simulink model "FlameAnalysis"  (R2015b)
settings: Solver=ode45  SolverMode=SingleTasking  StartTime=0.0  StopTime=1000  RelTol=1e-3
PreLoadFcn:
  | fprintf('loading now...\n')
PostLoadFcn:
  | model_name = gcs;
  | video_player_name=[model_name, '/From Multimedia File'];
  | video_path=get_param(video_player_name,'inputFileName');
  | model_path= get_param(model_name,'filename');
  | i=findstr('\',model_path);
  | 
  | if(~exist(video_path))
  |      video_path2=[model_path(1:i(end))  video_path(findstr('Video',video_path):end)];
  | 
  |      if(exist(video_path2))
  |           set_param(video_player_name,'inputFileName',video_path2);
  |      else
  |           j=findstr('\',video_path);
  |           video_path2=[model_path(1:i(end))  'Videos\' video_path(j(end)+1:end)];
  |           if(exist(video_path2))
  |                set_param(video_player_name,'inputFileName',video_path2);
  |           else
  |                avifiles=dir('videos\*.avi')
  |                set_param(video_player_name,'inputFileName',[model_path(1:i(end))  'Videos\'   avifiles(1).name]);
  |           end
  | 
  |      end
  | end
InitFcn:
  | clc
  | clear
  | global  t position wide dz_dt d2z_dt2 d3z_dt3 Af As dA_dt filePath Su_ Su alfa Karlovitz threshold model_name bords tWalls sheet model_path simulating numPointsAnalysis
  | simulating=true;
  | model_name = gcs;
  | model_path = [model_name, '/Edit Parameters'];
  | tbf = str2num(get_param(model_path,'tbf'));
  | ppcm= str2num(get_param(model_path,'ppcm'));
  | p2e= str2num(get_param(model_path,'p2e'));
  | 
  | nframes0= str2num(get_param(model_path,'nframes0'));
  | alfa= str2num(get_param(model_path,'alfa'));
  | fff= str2num(get_param(model_path,'fff'));
  | 
  | if((size(fff,2)~=1) & (size(fff,2)~=2))
  |     error('The flame front fraction must be scalar or 1x2-array');
  | end
  | order=str2num(get_param(model_path,'order'));
  | numberOfPoints=str2num(get_param(model_path,'numberOfPoints'));
  | orderAnalysis=str2num(get_param(model_path,'orderAnalysis'));
  | numPointsAnalysis=str2num(get_param(model_path,'numPointsAnalysis'));
  | uselog=str2num(get_param(model_path,'uselog'));
  | 
  | 
  | save2xls= strcmp('on',get_param(model_path,'save2xls'));
  | saveVideo= strcmp('on',get_param(model_path,'saveVideo'));
  | cfs= strcmp('on',get_param(model_path,'cfs'));
  | c3dv= strcmp('on',get_param(model_path,'c3dv'));
  | 
  | 
  | if(strcmp(get_param(model_path,'bge'),'Temporal Median Estimator'))
  |      bge=1;
  | elseif (strcmp(get_param(model_path,'bge'),'Temporal Median'))
  |     bge=2;
  |     bkgnd{1}=[gcs '/Background Estimator/Decomposing Red Movement/BG1/Temporal Median/Temporal Median'];
  |     bkgnd{2}=[gcs '/Background Estimator/Decomposing Green Movement/BG1/Temporal Median/Temporal Median'];
  |     bkgnd{3}=[gcs '/Background Estimator/Decomposing Blue Movement/BG1/Temporal Median/Temporal Median'];
  | 
  |     nframes0=max(nframes0,1);
  |     set_param([gcs '/Edit Parameters/'],'nframes0',num2str(nframes0));
  |     for i=1:3
  |         set_param(bkgnd{i}, 'tw', num2str(nframes0));
  |     end
  | else
  |     bge=3;
  | end
  | 
  | 
  | 
  | switch(get_param(model_path,'aprox_type'))
  |      case 'Profile'
  |            aprox_type=1;
  |            sheet='Profile';
  |      case 'Paraboloid (moving base)'
  |            aprox_type=2;
  |            sheet='Paraboloid';
  |      case 'Paraboloid(fixed base)'
  |            aprox_type=3;
  |            sheet='ParaboloidFB';
  |      case 'Spheroid'
  | ... (+19 lines)
StopFcn:
  | global editing  simulating
  | simulating = true;
  | try
  |       closeFunction
  | catch err
  |       simulating=false;
  |       err
  | end
  |   simulating=false;
model workspace (MATLAB code in the model file):
  | line_row =  22;
values from neighbouring files (symbols this model uses):
  m = size(BW,1)    [flameFront.m]    (also in putCircles.m = (y(i+1)-y(i))./(x(i+1)-x(i)))
  n = n(n==size(num,2)/4)    [averageOfVideos.m]    (also in countFramesOfVideo.m = 1; putCircles.m = length(y))
  vector = cast([row, col],'double')    [flameFront.m]
undefined symbols (not defined in the file or in its folder): strel
libraries: simulink x27, visionstatistics x14, visionconversions x9, visiontextngfix x9, visionmorphops x7, dspvision x4, visionsinks x2, visiongeotforms x1
(part 3 of 3)

== matlab function FlameAnalysis/Flame Front Estimation/Embedded MATLAB Function ==
  data: BW input; BBox input; Y output size=[2 (size(BW,1)*2 + size(BW,2)*2)*50] [0..1000000]; L output size=[1 size(BW,1)*100 ] [0..1000000]; fraction input; y_electrodes input; profile input; newBW output size=size(BW)
%Function that analyses a boolean image with a sylouette of a flame, and
%returns the coordinates of the upper border of the image and the vector
%necessary for ploting the image.
%PARAMETERS:
%   BW: Boolean Image with closed white profile
%   BBox: vector containing the dimensions of the box that encloses the
%   flame in the form BBox=[x1 y1 w1 h1]
%   Perimeter=Perimeter of the blob
%   fraction: a vector or scalar containing the fraction of the flame front
%       desired it can be either on the form: 0<fraction<=1 or fraction=[L R]
%       where 0<L,R<=1
%   aprox_type: indicates the kind of aproximation that will be ploted on the
%       image 
%           aprox_type=1:     Profile
%           aprox_type=2:     Paraboloid with moving base
%           aprox_type=3:     Paraboloid with fixed base
%           aprox_type=4:     Spheroid 
%           aprox_type=5:     Profile Spheroid 
%RETURNS:
%   Y: Coordinates of the upper border of the image independently from the
%       aprox_type, in the form Y=[x;y]
%   P: Coordinates of the upper border of the image depending on the
%       aprox_type, in the form L=[x1 y1 x2 y2 ... xn yn]
function [Y,L,newBW]=flameFront(BW,BBox,fraction, y_electrodes, profile)

m=size(BW,1);
Y=zeros(2,m*10);
L=zeros(1,m*20);
newBW=BW;
coder.extrinsic('flameFront');
if(numel(find(BW))>9)
    [Y,L,newBW]=flameFront(BW,BBox,fraction, y_electrodes, profile);
end

== matlab function FlameAnalysis/Display Results/Convertion to phisycal Data/Array To Scalar ==
  data: u input; position output; cmpf input; p2e input; wide output
function [position, wide] = array2scalar(u,cmpf,p2e)

position=double((u(1,1)+u(1,3)-p2e))*cmpf;
wide=u(1,4)*cmpf;
wide=wide;

== matlab function FlameAnalysis/Background Estimator/CompileBW ==
  data: I1 input; I2 input; I3 input; comparison output
function comparison  = compileRGB(I1,I2,I3)
[m,n]=size(I1);
comparison=zeros([m*4 n 3],'single');

coder.extrinsic('compileRGB');
[ comparison] = compileRGB(I1,I2,I3);

== matlab function FlameAnalysis/Background Estimator/MATLAB Function ==
  data: u input; y output
function y = fcn(u)
%#codegen

y = sum(u,3);

== matlab function FlameAnalysis/Background Estimator/Region filtering/blobDepurator ==
  data: areas input; blobs input; Y output size=[1 4]
function Y  =blobDepurator(areas,  blobs)

%Selection of the larger blobs that represent more than 50% of the total
%area.

[areas, i]=sort(areas,'descend');
blobs=blobs(i,:);



areatotal=sum(areas);

art=0;
 i=cast(0,'int32');
while(art/areatotal<=0.5)
    i=i+1;
    art=sum(areas(1:i));
end
%i=find(cumsum(areas)>0.5*sum(areas),1,'first');
areas(i+1:end)=0;
blobs(i+1:end,:)=0;


[A, i]=sort(blobs(:,1)+blobs(:,1),'descend');
Y=blobs(i(1),:);

== matlab function FlameAnalysis/Background Estimator/CompileBackground ==
  data: comparison output; I1 input; I2 input; I3 input; together output
function [comparison, together ]   = compileRGB(I1,I2,I3)
[m,n]=size(I1);
comparison=zeros([m*4 n 3],'single');
together=zeros([m n 3],'single');
coder.extrinsic('compileRGB');
[comparison, together ] = compileRGB(I1,I2,I3);

== matlab function FlameAnalysis/Background Estimator/CompileBackground1 ==
  data: I1 input; comparison output; I2 input; I3 input; together output
function [comparison, together ] = compileRGB(I1,I2,I3)
[m,n]=size(I1);
comparison=zeros([m*4 n 3],'single');
together=zeros([m n 3],'single');
coder.extrinsic('compileRGB');
[comparison, together ] = compileRGB(I1,I2,I3);

== matlab function FlameAnalysis/Display Results/Crop ==
  data: video input; y output; scissors input
function y = cropVideo(video,scissors)
%#codegen
y=zeros(size(video),'single');
scissors=cast(scissors,'logical');
j=[2 3 1];
for i=1:size(video,3)
    A1=video(:,:,i);
    A2=video(:,:,j(i));
    
    B=zeros(size(A1));
    B(~scissors)=A1(~scissors);
    B(scissors)=1-A2(scissors);        
    y(:,:,i)=B;
end

== matlab function FlameAnalysis/Background Estimator/Subsystem/fill1 ==
  data: I input; y output
function y = fcn2(I)
coder.extrinsic('imfill');
y=logical(zeros(size(I)));
y = logical(imfill(I,'holes'));

== matlab function FlameAnalysis/Background Estimator/Split Image ==
  data: imRGB input; R output; G output; B output
function [R,G,B]= breakRGBdown(imRGB)
%#codegen
coder.extrinsic('medfilt2');

R=imRGB(:,:,1);
G=imRGB(:,:,2);
B=imRGB(:,:,3);


R=medfilt2(R,[3 3]);
G=medfilt2(G,[3 3]);
B=medfilt2(B,[3 3]);
